simulink model "Project_The_Usual_Suspects"  (R2021a)
settings: Solver=VariableStepAuto  StartTime=0.0  StopTime=50  RelTol=1e-3
libraries: simulink x1
settings Model: Creator=DOLL  LastModifiedBy=DOLL

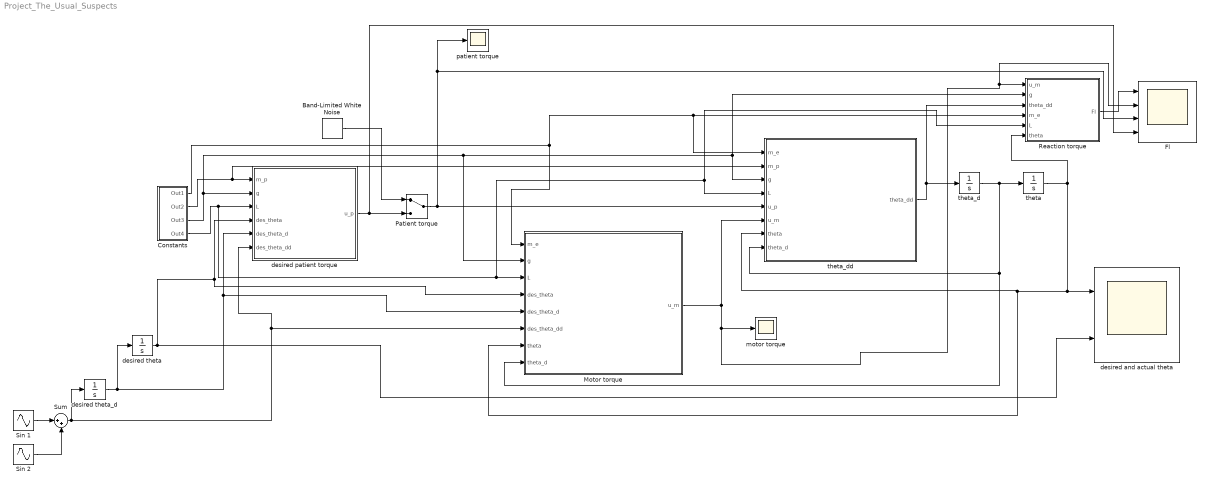
== system Project_The_Usual_Suspects ==
  Band-Limited White Noise : simulink/Sources/Band-Limited White Noise  Cov=[0.1]  Ts=0.1  seed=[23341]
  Constants : Subsystem
  Fl : Scope  NumInputPorts=4
  Motor torque : MATLAB Function  TreatAsAtomicUnit=on
  Patient torque : ManualSwitch
  Reaction torque : MATLAB Function  TreatAsAtomicUnit=on
  Sin 1 : Sin  Frequency=0.5  SampleTime=0
  Sin 2 : Sin  Phase=180  SampleTime=0
  Sum : Sum  Inputs=|++
  desired and actual theta : Scope  NumInputPorts=2
  desired patient torque : MATLAB Function  TreatAsAtomicUnit=on
  desired theta : Integrator
  desired theta_d : Integrator
  motor torque : Scope
  patient torque : Scope
  theta : Integrator
  theta_d : Integrator
  theta_dd : MATLAB Function  TreatAsAtomicUnit=on
  wires:
  desired theta/1 -> desired and actual theta/2, Motor torque/4(des_theta), desired patient torque/4(des_theta)
  desired theta_d/1 -> desired theta/1, desired patient torque/5(des_theta_d), Motor torque/5(des_theta_d)
  Constants/2(Out2) -> theta_dd/2(m_p), desired patient torque/1(m_p)
  Constants/3(Out3) -> Motor torque/2(g), theta_dd/3(g), Reaction torque/2(g), desired patient torque/2(g)
  Constants/4(Out4) -> Reaction torque/5(L), theta_dd/4(L), Motor torque/3(L), desired patient torque/3(L)
  desired patient torque/1(u_p) -> Fl/4, Patient torque/2
  Band-Limited White Noise/1 -> Patient torque/1
  Constants/1(Out1) -> Reaction torque/4(m_e), theta_dd/1(m_e), Motor torque/1(m_e)
  Motor torque/1(u_m) -> Fl/2, Reaction torque/1(u_m), motor torque/1, theta_dd/6(u_m)
  Patient torque/1 -> Fl/3, patient torque/1, theta_dd/5(u_p)
  theta_dd/1(theta_dd) -> theta_d/1, Reaction torque/3(theta_dd)
  theta_d/1 -> theta/1, Motor torque/8(theta_d), theta_dd/8(theta_d)
  theta/1 -> Reaction torque/6(theta), theta_dd/7(theta), Motor torque/7(theta), desired and actual theta/1
  Sum/1 -> desired theta_d/1, desired patient torque/6(des_theta_dd), Motor torque/6(des_theta_dd)
  Sin 1/1 -> Sum/1
  Sin 2/1 -> Sum/2
  Reaction torque/1(Fl) -> Fl/1

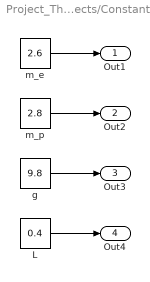
== system Project_The_Usual_Suspects/Constants ==
  L : Constant  Value=0.4
  g : Constant  Value=9.8
  m_e : Constant  Value=2.6
  m_p : Constant  Value=2.8
  Out1 : Outport
  Out2 : Outport  Port=2
  Out3 : Outport  Port=3
  Out4 : Outport  Port=4
  wires:
  g/1 -> Out3/1
  L/1 -> Out4/1
  m_p/1 -> Out2/1
  m_e/1 -> Out1/1

== matlab function Project_The_Usual_Suspects/Motor torque ==
  data: m_e input; u_m output; g input; L input; des_theta input; des_theta_d input; des_theta_dd input; theta input; theta_d input
function u_m = fcn(m_e, g, L, des_theta, des_theta_d, des_theta_dd, theta, theta_d)
K = 13;
D = 25;
J_e = 0.04; %m_e*L^2/3;
G_e = m_e*g*L*sin(theta)/2;
C_e = 0;

u_m = K*(des_theta-theta) + D*(des_theta_d-theta_d) + J_e*des_theta_dd + C_e*theta_d + G_e;

== matlab function Project_The_Usual_Suspects/desired patient torque ==
  data: m_p input; g input; u_p output; L input; des_theta input; des_theta_d input; des_theta_dd input
function u_p = fcn(m_p, g, L, des_theta, des_theta_d, des_theta_dd)
J_p = 0.036; %m_p*L^2/3;
G_p = m_p*g*L*sin(des_theta)/2;
C_p = 0;
u_p = J_p*des_theta_dd + C_p*des_theta_d + G_p;

== matlab function Project_The_Usual_Suspects/theta_dd ==
  data: m_e input; theta_dd output; m_p input; g input; L input; u_p input; u_m input; theta input; theta_d input
function theta_dd = fcn(m_e, m_p, g, L, u_p, u_m, theta, theta_d)
J_e = 0.04; %m_e*L^2/3;
J_p = 0.036; %m_p*L^2/3;
C_e = 0;
C_p = 0;
G_e = m_e*g*L*sin(theta)/2;
G_p = m_p*g*L*sin(theta)/2;
theta_dd = (u_m + u_p - (C_e+C_p)*theta_d - (G_e+G_p))/(J_e+J_p);

== matlab function Project_The_Usual_Suspects/Reaction torque ==
  data: u_m input; Fl output; g input; theta_dd input; m_e input; L input; theta input
function Fl = fcn(u_m, g, theta_dd, m_e, L, theta)
J_e = 0.04;
G_e = m_e*g*L*sin(theta)/2;
Fl = u_m - G_e - (J_e*theta_dd);
